simulink model "simulink7"  (R2025b)
settings: Solver=VariableStepAuto  StartTime=0.0  StopTime=1.5  RelTol=1e-3
settings Model: Creator=kl247  LastModifiedBy=kl247

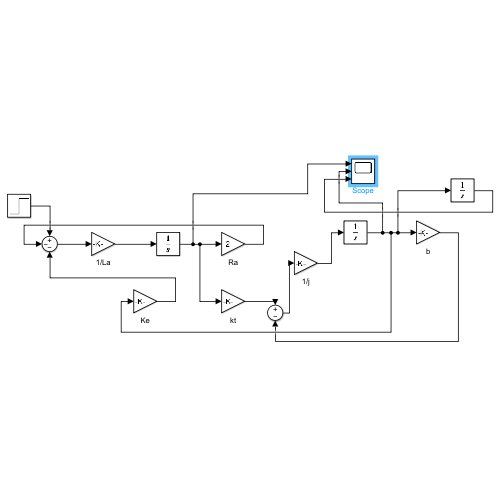
[thumbnail: Simulink's stored preview of the top-level diagram]
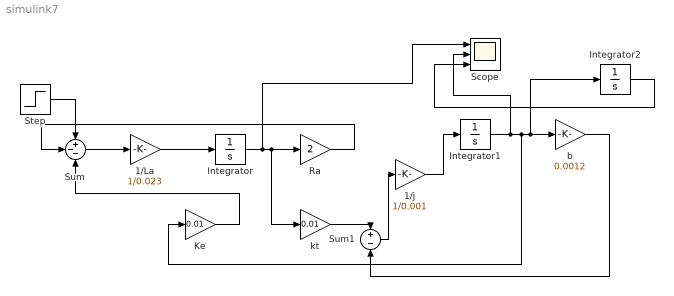
== system simulink7 ==
  1/La : Gain  Gain=1/0.023
  1/j : Gain  Gain=1/0.001
  Integrator : Integrator
  Integrator1 : Integrator
  Integrator2 : Integrator
  Ke : Gain  Gain=0.01
  Ra : Gain  Gain=2
  Scope : Scope  NumInputPorts=3
      settings: ActiveDisplayYMinimum=-0.74721817775340427  ActiveDisplayYMaximum=6.7249635997806392
  Step : Step  Time=0  After=12  SampleTime=0
  Sum : Sum  Inputs=+--
  Sum1 : Sum  Inputs=+-
  b : Gain  Gain=0.0012
  kt : Gain  Gain=0.01
  wires:
  Step/1 -> Sum/1
  Sum/1 -> 1/La/1
  1/La/1 -> Integrator/1
  Integrator/1 -> Scope/1, kt/1, Ra/1
  Ra/1 -> Sum/2
  kt/1 -> Sum1/1
  Sum1/1 -> 1/j/1
  1/j/1 -> Integrator1/1
  Integrator1/1 -> Scope/2, Ke/1, Integrator2/1, b/1
  b/1 -> Sum1/2
  Ke/1 -> Sum/3
  Integrator2/1 -> Scope/3
